simulink model "Simulink_VDP_nlMPC"  (R2022a)
settings: Solver=FixedStepAuto  StartTime=0.0  StopTime=Tf  FixedStep=Ts  RelTol=1e-3
values from neighbouring files (symbols this model uses):
  D = zeros(size(Z,1),size(U,1))    [VanDerPol_MPC_Koopman.m]
  Ts = 1e-2    (= 0.01)    [VanDerPol_MPC.m]
libraries: mpclib x1
settings Model: Creator=sergiovaneg  LastModifiedBy=sergiovaneg

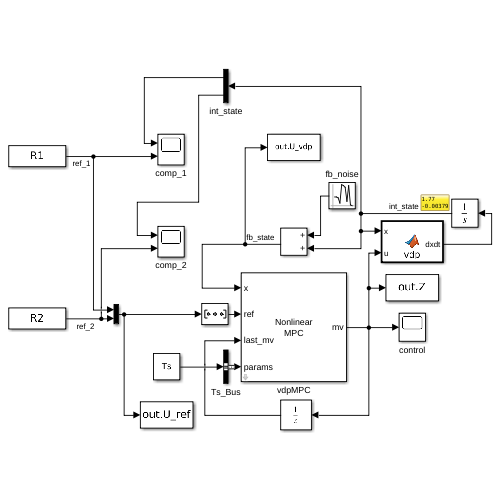
[thumbnail: Simulink's stored preview of the top-level diagram]
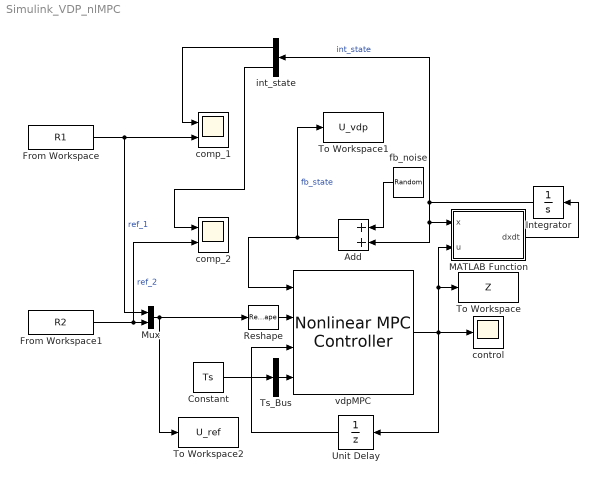
== system Simulink_VDP_nlMPC ==
  Add : Sum
  Constant : Constant  Value=Ts
  From Workspace : FromWorkspace  VariableName=R1
  From Workspace1 : FromWorkspace  VariableName=R2
  Integrator : Integrator  InitialCondition=[0;0]
  MATLAB Function : MATLAB Function  TreatAsAtomicUnit=on
  Mux : Mux  Inputs=2
  Reshape : Reshape  OutputDimensionality=Row vector (2-D)
  To Workspace : ToWorkspace  VariableName=Z  SampleTime=Ts
      settings: Save2DSignal=2-D array (concatenate along first dimension)
  To Workspace1 : ToWorkspace  VariableName=U_vdp  SampleTime=Ts
      settings: Save2DSignal=2-D array (concatenate along first dimension)
  To Workspace2 : ToWorkspace  VariableName=U_ref  SampleTime=Ts
      settings: Save2DSignal=2-D array (concatenate along first dimension)
  Ts_Bus : BusCreator  Inputs=1  OutDataTypeStr=Bus: Ts_Bus  NonVirtualBus=on
      settings: InheritFromInputs=off
  Unit Delay : UnitDelay  SampleTime=-1  HasFrameUpgradeWarning=on
  comp_1 : Scope  NumInputPorts=2
  comp_2 : Scope  NumInputPorts=2
  control : Scope
  fb_noise : RandomNumber  Variance=0.001  Seed=[2;3]  SampleTime=Ts
  int_state : Demux  Outputs=2
  vdpMPC : mpclib/Nonlinear MPC Controller  nlmpcobj=nlobj  UseObjectTs=on  UseMEX=off  md_enabled=off  mvtarget_enabled=off  param_enabled=on  cost_enabled=off  mvseq_enabled=off  stateseq_enabled=off  ovseq_enabled=off  slack_enabled=off  status_enabled=off  ov_min=off  ov_max=off  mv_min=off  mv_max=off  mvrate_min=off  mvrate_max=off  state_min=off  state_max=off  ov_weight=off  mv_weight=off  mvrate_weight=off  ecr_weight=off  nlp_initialize=off
  wires:
  Add/1 -> To Workspace1/1, vdpMPC/1  "fb_state"
  From Workspace/1 -> comp_1/2, Mux/1  "ref_1"
  int_state/1 -> comp_1/1
  fb_noise/1 -> Add/1
  Reshape/1 -> vdpMPC/2
  vdpMPC/1 -> MATLAB Function/2(u), To Workspace/1, Unit Delay/1, control/1
  Constant/1 -> Ts_Bus/1
  Integrator/1 -> int_state/1, Add/2, MATLAB Function/1(x)  "int_state"
  From Workspace1/1 -> comp_2/2, Mux/2  "ref_2"
  Unit Delay/1 -> vdpMPC/3
  int_state/2 -> comp_2/1
  MATLAB Function/1(dxdt) -> Integrator/1
  Mux/1 -> To Workspace2/1, Reshape/1
  Ts_Bus/1 -> vdpMPC/4

== matlab function Simulink_VDP_nlMPC/MATLAB Function ==
  data: x input; u input; dxdt output
function dxdt = vdp(x,u)
    dxdt = zeros(2,1);
    dxdt(1) = 2*x(2);
    dxdt(2) = -0.8*x(1)+2*x(2)-10*(x(1)^2)*x(2)+u;
